simulink model "AVP_Main"  (R2018b)
settings: Solver=FixedStepDiscrete  StartTime=0.0  StopTime=inf  FixedStep=0.01  RelTol=1e-3
PostLoadFcn:
  | if any(exist('dsrtsu_mdlpostloadfcn', 'file') ~= 0), dsrtsu_mdlpostloadfcn('Execute', bdroot); end
settings Model: DSRTSU_INTERNAL_RTI_VER=540  DSRTSU_INTERNAL_RTI_TYPE=rti1401  RTICANMMDATA=struct('GeneralSetupData',struct('modelroot','D:\0001_SAIC_MBD\03_ZOP\ZOP_Integration\ZOP_Integration_AVP','generalsettings',struct('filesettings',struct('destfolder',struct('Name','RTICANMM_FILES','Check',1),'buildfolder',struct('Name','.','Check',1),'AbsDestfolder',struct('Name','D:\0001_SAIC_MBD\03_ZOP\ZOP_Integration\ZOP_Integration_AVP\RTICANMM_FILES'),'AbsBuildfolder',struct('Name','D:\0001_SAIC_MBD\03_ZOP\ZOP_Integration\ZOP_Integration_AVP'))),'options',struct('addpaths',1,'rmpaths',1,'addtrcexclusion',logical(1),'cannavigator',struct('checkmonitoring',0),'show_usrtrc',0,'use_usrtrc',0),'advanced',struct('options',ones(1,100)),'MPSetup',{{}},'RTI',struct('Type','RTI1401','Ver','7.12','Date','02-May-2019'),'modelname','AVP_Main','block','AVP_Main'))  DSRTSU_INTERNAL_RTIFPGA=130  Creator=chenx  LastModifiedBy=qiand
settings OptimizationCC: BlockReduction=off  ConditionallyExecuteInputs=off  DefaultUnderspecifiedDataType=single  BufferReuse=off  EnhancedBackFolding=on  ExpressionFolding=off  PassReuseOutputArgsThreshold=0  LocalBlockOutputs=off  OptimizeBlockOrder=speed  DifferentSizesBufferReuse=on
settings DebuggingCC: ParameterTunabilityLossMsg=error  UnderSpecifiedDimensionMsg=warning
settings HardwareCC: ProdBitPerPointer=32  ProdBitPerSizeT=32  ProdBitPerPtrDiffT=32  ProdLargestAtomicInteger=Integer  ProdEndianess=BigEndian  ProdWordSize=32  ProdHWDeviceType=Custom Processor->Custom  TargetIntDivRoundTo=Zero  TargetEndianess=BigEndian  TargetHWDeviceType=Custom Processor->Custom
settings ModelReferenceCC: ModelReferenceNumInstancesAllowed=Single
settings SFSimCC: MATLABDynamicMemAlloc=off
settings RTWCC: SystemTargetFile=rti1401.tlc  MakeCommand=make_rti  TemplateMakefile=rti1401.tmf  Description=dSPACE DS1401 Hardware Platform  GenerateReport=on  LaunchReport=on
settings CodeAppCC: OperatorAnnotations=on
settings STFCustomTargetCC: ParMdlRefBuildCompliant=on  SystemTargetFile=rti1401.tlc
settings GRTTargetCC: TargetLangStandard=C89/C90 (ANSI)  CompOptLevelCompliant=off  ConcurrentExecutionCompliant=off  CombineOutputUpdateFcns=off  MatFileLogging=off  CPPClassGenCompliant=off  UseToolchainInfoCompliant=off

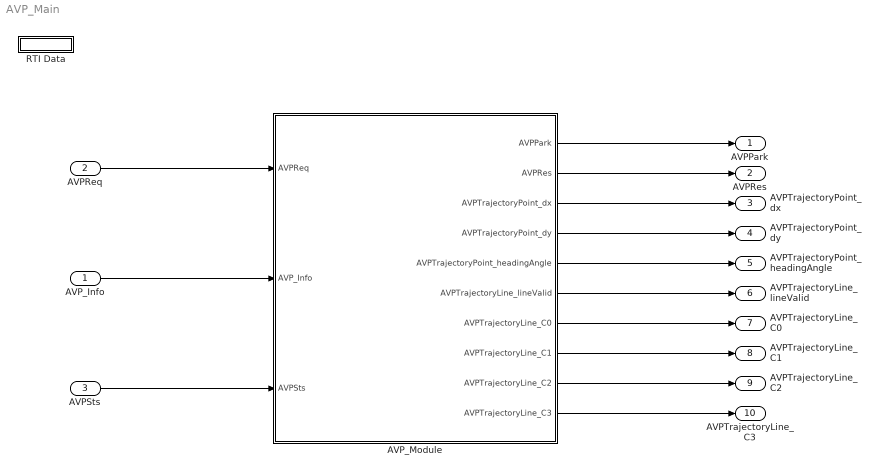
== system AVP_Main ==
  AVP_Info : Inport  OutDataTypeStr=Bus: AVP_OUTPUT_ST  BusOutputAsStruct=on
  AVPReq : Inport  Port=2  OutDataTypeStr=uint8
  AVPSts : Inport  Port=3  OutDataTypeStr=uint8
  AVP_Module : Subsystem
  RTI Data : Subsystem  Tag=struct('RTIDataServer',struct('RTIDataServerVs','2','RTIModelDescription','struct(''main'',''AVP_Main'',''sub'',''AVP_Main'',''isMp'',0)'))  LoadFcn="if exist('rtidc'), try,  rtidc('DataHostBlockClbLoad', gcbh); catch, disp(['Warning: ''LoadFcn'' for RTI Data block failed: ' lasterr]); end, end,"  mask(RTI_DATA_HOST){}
      mask help:
      | RTI Data Block.
      | This block is used by RTI to store internal model-dependent data.
      | Please keep this block on the root level of the model. Deleting this block will result in data loss.
      |
      | NEVER DELETE OR COPY THIS BLOCK!
      settings: CopyFcn="if exist('rtidc'), try,  rtidc('DataHostBlockClbCopy', gcbh); catch, disp(['Warning: ''CopyFcn'' for RTI Data block failed: ' lasterr]); end, end,"  DeleteFcn="if exist('rtidc'), try,  rtidc('DataHostBlockClbDelete', gcbh); catch, disp(['Warning: ''DeleteFcn'' for RTI Data block failed: ' lasterr]); end, end,"  ModelCloseFcn="if exist('rtidc'), try,  rtidc('DataHostBlockClbModelClose', gcbh); catch, disp(['Warning: ''ModelCloseFcn'' for RTI Data block failed: ' lasterr]); end, end,"  PreSaveFcn="if exist('rtidc'), try,  rtidc('DataHostBlockClbPreSave', gcbh); catch, disp(['Warning: ''PreSaveFcn'' for RTI Data block failed: ' lasterr]); end, end,"  PostSaveFcn="if exist('rtidc'), try,  rtidc('DataHostBlockClbPostSave', gcbh); catch, disp(['Warning: ''PostSaveFcn'' for RTI Data block failed: ' lasterr]); end, end,"  NameChangeFcn="if exist('rtidc'), try,  rtidc('DataHostBlockClbNameChange', gcbh); catch, disp(['Warning: ''NameChangeFcn'' for RTI Data block failed: ' lasterr]); end, end,"
      mask Help:
      | RTI Data Block.
      | This block is used by RTI to store internal model-dependent data.
      | Please keep this block on the root level of the model. Deleting this block will result in data loss.
      | 
      | NEVER DELETE OR COPY THIS BLOCK!
      mask Display:
      | text(0.5, 0.5, 'RTI Data', 'HorizontalAlignment', 'center');
      | plot([1 0]);
  AVPPark : Outport  OutDataTypeStr=uint8
  AVPRes : Outport  Port=2  OutDataTypeStr=uint8
  AVPTrajectoryPoint_dx : Outport  Port=3
  AVPTrajectoryPoint_dy : Outport  Port=4
  AVPTrajectoryPoint_headingAngle : Outport  Port=5
  AVPTrajectoryLine_lineValid : Outport  Port=6  OutDataTypeStr=boolean
  AVPTrajectoryLine_C0 : Outport  Port=7
  AVPTrajectoryLine_C1 : Outport  Port=8
  AVPTrajectoryLine_C2 : Outport  Port=9
  AVPTrajectoryLine_C3 : Outport  Port=10
  wires:
  AVP_Info/1 -> AVP_Module/2(AVP_Info)
  AVPReq/1 -> AVP_Module/1(AVPReq)
  AVPSts/1 -> AVP_Module/3(AVPSts)
  AVP_Module/1(AVPPark) -> AVPPark/1
  AVP_Module/2(AVPRes) -> AVPRes/1
  AVP_Module/3(AVPTrajectoryPoint_dx) -> AVPTrajectoryPoint_dx/1
  AVP_Module/4(AVPTrajectoryPoint_dy) -> AVPTrajectoryPoint_dy/1
  AVP_Module/7(AVPTrajectoryLine_C0) -> AVPTrajectoryLine_C0/1
  AVP_Module/8(AVPTrajectoryLine_C1) -> AVPTrajectoryLine_C1/1
  AVP_Module/9(AVPTrajectoryLine_C2) -> AVPTrajectoryLine_C2/1
  AVP_Module/10(AVPTrajectoryLine_C3) -> AVPTrajectoryLine_C3/1
  AVP_Module/6(AVPTrajectoryLine_lineValid) -> AVPTrajectoryLine_lineValid/1
  AVP_Module/5(AVPTrajectoryPoint_headingAngle) -> AVPTrajectoryPoint_headingAngle/1

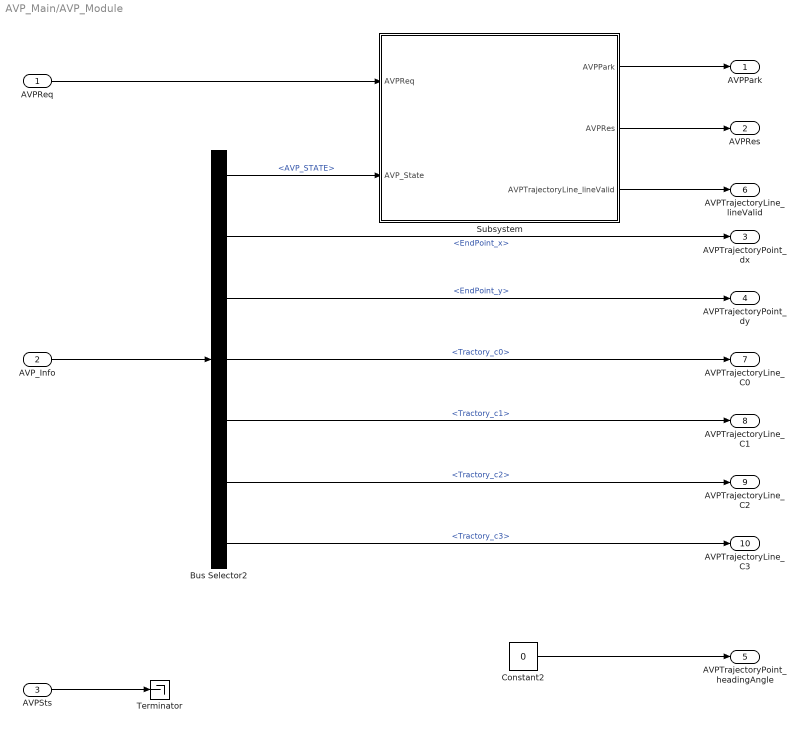
== system AVP_Main/AVP_Module ==
  AVPReq : Inport  OutDataTypeStr=uint8
  AVP_Info : Inport  Port=2  OutDataTypeStr=Bus: AVP_OUTPUT_ST
  AVPSts : Inport  Port=3  OutDataTypeStr=uint8
  Bus Selector2 : BusSelector  OutputSignals=AVP_STATE,EndPoint_x,EndPoint_y,Tractory_c0,Tractory_c1,Tractory_c2,Tractory_c3
  Constant2 : Constant  Value=0
  Subsystem : Subsystem
  Terminator : Terminator
  AVPPark : Outport  OutDataTypeStr=uint8
  AVPRes : Outport  Port=2  OutDataTypeStr=uint8
  AVPTrajectoryPoint_dx : Outport  Port=3
  AVPTrajectoryPoint_dy : Outport  Port=4
  AVPTrajectoryPoint_headingAngle : Outport  Port=5
  AVPTrajectoryLine_lineValid : Outport  Port=6  OutDataTypeStr=boolean
  AVPTrajectoryLine_C0 : Outport  Port=7
  AVPTrajectoryLine_C1 : Outport  Port=8
  AVPTrajectoryLine_C2 : Outport  Port=9
  AVPTrajectoryLine_C3 : Outport  Port=10
  wires:
  AVP_Info/1 -> Bus Selector2/1
  AVPSts/1 -> Terminator/1
  AVPReq/1 -> Subsystem/1(AVPReq)
  Subsystem/3(AVPTrajectoryLine_lineValid) -> AVPTrajectoryLine_lineValid/1
  Constant2/1 -> AVPTrajectoryPoint_headingAngle/1
  Subsystem/2(AVPRes) -> AVPRes/1
  Subsystem/1(AVPPark) -> AVPPark/1
  Bus Selector2/1 -> Subsystem/2(AVP_State)  "<AVP_STATE>"
  Bus Selector2/2 -> AVPTrajectoryPoint_dx/1  "<EndPoint_x>"
  Bus Selector2/3 -> AVPTrajectoryPoint_dy/1  "<EndPoint_y>"
  Bus Selector2/4 -> AVPTrajectoryLine_C0/1  "<Tractory_c0>"
  Bus Selector2/5 -> AVPTrajectoryLine_C1/1  "<Tractory_c1>"
  Bus Selector2/6 -> AVPTrajectoryLine_C2/1  "<Tractory_c2>"
  Bus Selector2/7 -> AVPTrajectoryLine_C3/1  "<Tractory_c3>"

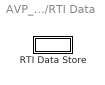
== system AVP_Main/RTI Data ==
  RTI Data Store : Subsystem  Tag="struct('private',struct('version',struct('dsVer',uint32(2),'dsVerCreation',uint32(2),'RTI',struct('ver','7.12','type','RTI1401')),'access',struct('type','Model','isPerm',1,'created',['11-Dec-2020 17:36:09'],'modified',['17-Mar-2021 15:49:09'],'location','')),'public',struct('main',struct('data',[]),'sub',struct('name',{{'AVP_Main'}},'data',{{struct('TH',struct('thTaskInfo',struct('taskType',{'TIMER','HWINT','TMRINT','SWINT','GLINT'},'tasksNumOf',{1,0,0,0,0},'srcIds',{{'TIMERA'},{},{},{},{}},'taskNames',{{['Timer Task 1']},{},{},{},{}})),'th_tc',struct('dataType','TASK','taskGroupId','','taskGroupList',{{}},'taskSchedulingPolicy','FCFS','taskType','TIMER','blkh',-1,'srcId','TIMERA','srcSgnName',['Timer A interrupt'],'srcCpuName','','taskName',['Timer Task 1  [0.01] s'],'taskNameDisplayExt','','smplTime',0.01,'smplTimeOffs',0,'hasFixedPriority',0,'priority',1,'hasFixedOvc',0,'ovcType',1,'ovcMax',1),'tc_th',struct('dataType','TASK','taskGroupId','','taskGroupList',{{}},'taskSchedulingPolicy','FCFS','taskType','TIMER','blkh',-1,'srcId','TIMERA','srcSgnName',['Timer A interrupt'],'srcCpuName','','taskName',['Timer Task 1  [0.01] s'],'taskNameDisplayExt','','smplTime',0.01,'smplTimeOffs',0,'hasFixedPriority',0,'priority',1,'hasFixedOvc',0,'ovcType',1,'ovcMax',1))}})))"  mask(RTI_DATA_STORE){}
      mask help:
      | RTI Data Store Block. This block is used by RTI to store internal model dependent data. Deleting this block will result in data loss.
      |
      | NEVER DELETE, COPY, OR MODIFY THIS BLOCK!
      mask Help:
      | RTI Data Store Block. This block is used by RTI to store internal model dependent data. Deleting this block will result in data loss.
      | 
      | NEVER DELETE, COPY, OR MODIFY THIS BLOCK!
      mask Display: text(0.5, 0.5, ' ', 'HorizontalAlignment', 'center');

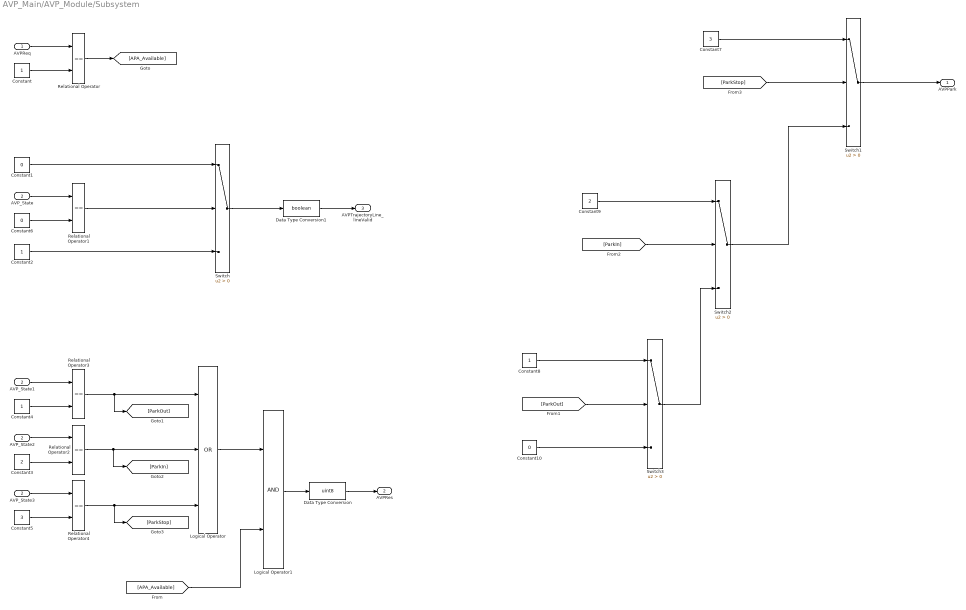
== system AVP_Main/AVP_Module/Subsystem ==
  AVPReq : Inport  OutDataTypeStr=uint8
  AVP_State : Inport  Port=2
  AVP_State1 : InportShadow  Port=2
  AVP_State2 : InportShadow  Port=2
  AVP_State3 : InportShadow  Port=2
  Constant{,2,4,8} (4 alike) : Constant  OutDataTypeStr=uint8
  Constant1 : Constant  Value=0  OutDataTypeStr=uint8
  Constant10 : Constant  Value=0  OutDataTypeStr=uint8
  Constant3 : Constant  Value=2  OutDataTypeStr=uint8
  Constant5 : Constant  Value=3  OutDataTypeStr=uint8
  Constant6 : Constant  Value=0  OutDataTypeStr=uint8
  Constant7 : Constant  Value=3  OutDataTypeStr=uint8
  Constant9 : Constant  Value=2  OutDataTypeStr=uint8
  Data Type Conversion : DataTypeConversion  OutDataTypeStr=uint8
  Data Type Conversion1 : DataTypeConversion  OutDataTypeStr=boolean
  Logical Operator : Logic  Operator=OR  Inputs=3  AllPortsSameDT=off  OutDataTypeStr=boolean
  Logical Operator1 : Logic  AllPortsSameDT=off  OutDataTypeStr=boolean
  Relational Operator{,1..4} (5 alike) : RelationalOperator  Operator===  OutDataTypeStr=boolean  RndMeth=Simplest
  Switch{,1..3} (4 alike) : Switch  Criteria=u2 > Threshold
  AVPPark : Outport  OutDataTypeStr=uint8
  AVPRes : Outport  Port=2  OutDataTypeStr=uint8
  AVPTrajectoryLine_lineValid : Outport  Port=3  OutDataTypeStr=boolean
  wires:
  Constant/1 -> Relational Operator/2
  Relational Operator/1 -> [APA_Available]
  AVPReq/1 -> Relational Operator/1
  AVP_State/1 -> Relational Operator1/1
  Constant6/1 -> Relational Operator1/2
  Relational Operator1/1 -> Switch/2
  Constant1/1 -> Switch/1
  Switch/1 -> Data Type Conversion1/1
  Constant2/1 -> Switch/3
  Constant3/1 -> Relational Operator2/2
  Constant4/1 -> Relational Operator3/2
  AVP_State1/1 -> Relational Operator3/1
  AVP_State2/1 -> Relational Operator2/1
  Constant5/1 -> Relational Operator4/2
  AVP_State3/1 -> Relational Operator4/1
  Relational Operator3/1 -> [ParkOut], Logical Operator/1
  Relational Operator2/1 -> [ParkIn], Logical Operator/2
  Relational Operator4/1 -> [ParkStop], Logical Operator/3
  Logical Operator/1 -> Logical Operator1/1
  [APA_Available] -> Logical Operator1/2
  Logical Operator1/1 -> Data Type Conversion/1
  Constant7/1 -> Switch1/1
  Switch1/1 -> AVPPark/1
  [ParkStop] -> Switch1/2
  Switch2/1 -> Switch1/3
  [ParkIn] -> Switch2/2
  [ParkOut] -> Switch3/2
  Switch3/1 -> Switch2/3
  Constant8/1 -> Switch3/1
  Constant9/1 -> Switch2/1
  Constant10/1 -> Switch3/3
  Data Type Conversion/1 -> AVPRes/1
  Data Type Conversion1/1 -> AVPTrajectoryLine_lineValid/1

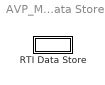
== system AVP_Main/RTI Data/RTI Data Store ==
  RTI Data Store : Subsystem  mask(RTI_DATA_STORE){}
      mask help:
      | RTI Data Store Block. This block is used by RTI to store internal model dependent data. Deleting this block will result in data loss.
      |
      | NEVER DELETE, COPY, OR MODIFY THIS BLOCK!
      mask Help:
      | RTI Data Store Block. This block is used by RTI to store internal model dependent data. Deleting this block will result in data loss.
      | 
      | NEVER DELETE, COPY, OR MODIFY THIS BLOCK!
      mask Display: text(0.5, 0.5, ' ', 'HorizontalAlignment', 'center');

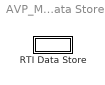
== system AVP_Main/RTI Data/RTI Data Store/RTI Data Store ==
  RTI Data Store : Subsystem  mask(RTI_DATA_STORE){}
      mask help:
      | RTI Data Store Block. This block is used by RTI to store internal model dependent data. Deleting this block will result in data loss.
      |
      | NEVER DELETE, COPY, OR MODIFY THIS BLOCK!
      mask Help:
      | RTI Data Store Block. This block is used by RTI to store internal model dependent data. Deleting this block will result in data loss.
      | 
      | NEVER DELETE, COPY, OR MODIFY THIS BLOCK!
      mask Display: text(0.5, 0.5, ' ', 'HorizontalAlignment', 'center');

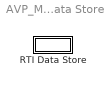
== system AVP_Main/RTI Data/RTI Data Store/RTI Data Store/RTI Data Store ==
  RTI Data Store : Subsystem  mask(RTI_DATA_STORE){}
      mask help:
      | RTI Data Store Block. This block is used by RTI to store internal model dependent data. Deleting this block will result in data loss.
      |
      | NEVER DELETE, COPY, OR MODIFY THIS BLOCK!
      mask Help:
      | RTI Data Store Block. This block is used by RTI to store internal model dependent data. Deleting this block will result in data loss.
      | 
      | NEVER DELETE, COPY, OR MODIFY THIS BLOCK!
      mask Display: text(0.5, 0.5, ' ', 'HorizontalAlignment', 'center');

== system AVP_Main/RTI Data/RTI Data Store/RTI Data Store/RTI Data Store/RTI Data Store ==
